simulink model "FIR_Filter_Reference"  (R2020b)
settings: Solver=VariableStepAuto  StartTime=0.0  StopTime=10.0  RelTol=1e-3
settings Model: Creator=Shirish  LastModifiedBy=Shirish
settings DataIOCC: SaveOutput=off  SaveTime=off

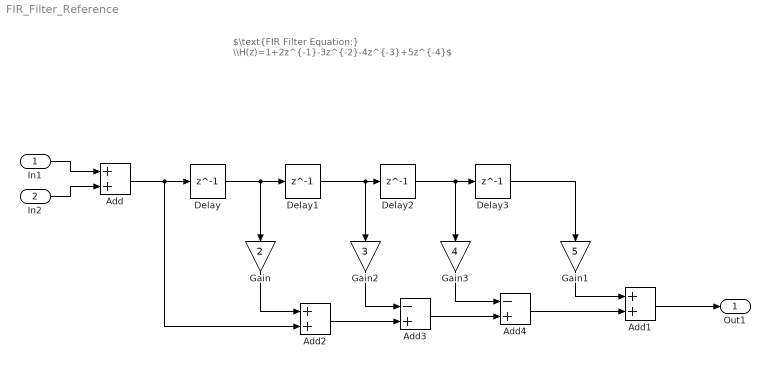
== system FIR_Filter_Reference ==
  note: $\text{FIR Filter Equation:} \\H(z)=1+2z^{-1}-3z^{-2}-4z^{-3}+5z^{-4}$
  In1 : Inport  OutDataTypeStr=double  PortDimensions=1  SampleTime=0
  In2 : Inport  Port=2  OutDataTypeStr=double  PortDimensions=1  SampleTime=0
  Add : Sum
  Add1 : Sum
  Add2 : Sum
  Add3 : Sum  Inputs=-+
  Add4 : Sum  Inputs=-+
  Delay{,1..3} (4 alike) : Delay  DelayLength=1
  Gain : Gain  Gain=2
  Gain1 : Gain  Gain=5
  Gain2 : Gain  Gain=3
  Gain3 : Gain  Gain=4
  Out1 : Outport  OutDataTypeStr=double  PortDimensions=1  SampleTime=0
  wires:
  Add4/1 -> Add1/2
  Gain/1 -> Add2/1
  Delay/1 -> Delay1/1, Gain/1
  Add/1 -> Delay/1, Add2/2
  Delay1/1 -> Delay2/1, Gain2/1
  Add3/1 -> Add4/2
  Gain3/1 -> Add4/1
  Delay2/1 -> Delay3/1, Gain3/1
  Gain2/1 -> Add3/1
  Add2/1 -> Add3/2
  In1/1 -> Add/1
  Delay3/1 -> Gain1/1
  Gain1/1 -> Add1/1
  In2/1 -> Add/2
  Add1/1 -> Out1/1
